simulink model "simulink_model"  (R2023b)
settings: Solver=ode23t  StartTime=0.0  StopTime=2  MaxStep=2e-5  RelTol=1e-3
undefined symbols (not defined in the file or in its folder): J, L_a, M_nom, Psi_nom, R_a, U_nom
settings Model: Creator=deniskirbaba  LastModifiedBy=deniskirbaba

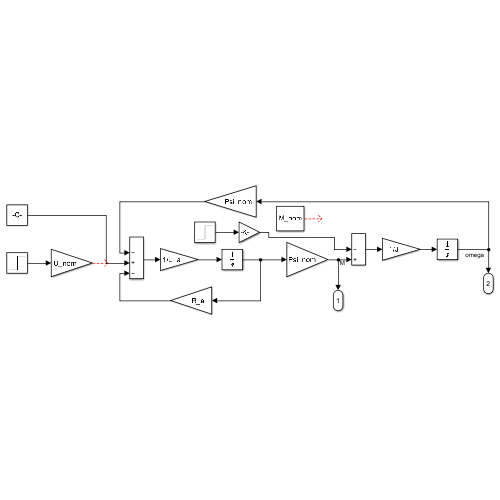
[thumbnail: Simulink's stored preview of the top-level diagram]
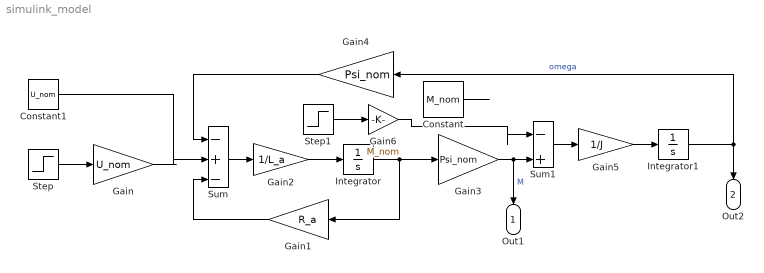
== system simulink_model ==
  Constant : Constant  Value=M_nom
  Constant1 : Constant  Value=U_nom
  Gain : Gain  Gain=U_nom
  Gain1 : Gain  Gain=R_a
  Gain2 : Gain  Gain=1/L_a
  Gain3 : Gain  Gain=Psi_nom
  Gain4 : Gain  Gain=Psi_nom
  Gain5 : Gain  Gain=1/J
  Gain6 : Gain  Gain=M_nom
  Integrator : Integrator
  Integrator1 : Integrator
  Step : Step  Before=0.5  SampleTime=0
  Step1 : Step  Before=0.5  SampleTime=0
  Sum : Sum  Inputs=|-+-
  Sum1 : Sum  Inputs=|-+
  Out1 : Outport
  Out2 : Outport  Port=2
  wires:
  Step/1 -> Gain/1
  Gain/1 -> ?
  Gain1/1 -> Sum/3
  Sum/1 -> Gain2/1
  Gain2/1 -> Integrator/1
  Integrator/1 -> Gain1/1, Gain3/1
  Gain4/1 -> Sum/1
  Gain3/1 -> Out1/1, Sum1/2  "M"
  Constant/1 -> ?
  Sum1/1 -> Gain5/1
  Gain5/1 -> Integrator1/1
  Integrator1/1 -> Gain4/1, Out2/1  "omega"
  Constant1/1 -> Sum/2
  Gain6/1 -> Sum1/1
  Step1/1 -> Gain6/1
